simulink model "g"  (R2018b)
settings: Solver=FixedStepAuto  StartTime=0.0  StopTime=10.68  FixedStep=0.01  RelTol=1e-3
settings Model: Creator=yizha  LastModifiedBy=yizha

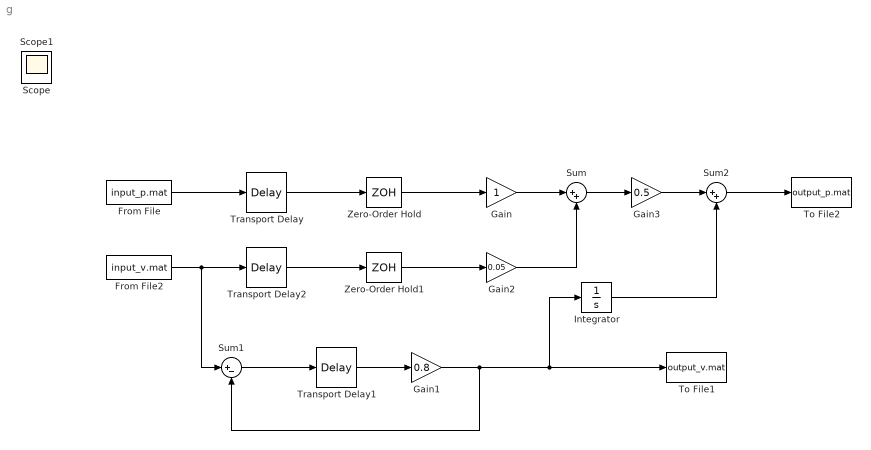
== system g ==
  From File : FromFile  FileName=input_p.mat  SampleTime=0
  From File2 : FromFile  FileName=input_v.mat  SampleTime=0
  Gain : Gain
  Gain1 : Gain  Gain=0.8
  Gain2 : Gain  Gain=0.05
  Gain3 : Gain  Gain=0.5
  Integrator : Integrator
  Sum : Sum  Inputs=|++
  Sum1 : Sum  Inputs=|+-
  Sum2 : Sum  Inputs=|++
  To File1 : ToFile  Filename=output_v.mat
  To File2 : ToFile  Filename=output_p.mat
  Transport Delay : TransportDelay  DelayTime=0.1
  Transport Delay1 : TransportDelay  DelayTime=0.1
  Transport Delay2 : TransportDelay  DelayTime=0.1
  Zero-Order Hold : ZeroOrderHold  SampleTime=0.1
  Zero-Order Hold1 : ZeroOrderHold  SampleTime=0.1
  Scope : Scope
  Scope1 : Scope
  wires:
  Sum1/1 -> Transport Delay1/1
  Transport Delay1/1 -> Gain1/1
  Gain1/1 -> Sum1/2, Integrator/1, To File1/1
  From File2/1 -> Sum1/1, Transport Delay2/1
  Transport Delay/1 -> Zero-Order Hold/1
  Gain/1 -> Sum/1
  Zero-Order Hold1/1 -> Gain2/1
  From File/1 -> Transport Delay/1
  Zero-Order Hold/1 -> Gain/1
  Transport Delay2/1 -> Zero-Order Hold1/1
  Gain2/1 -> Sum/2
  Sum2/1 -> To File2/1
  Integrator/1 -> Sum2/2
  Sum/1 -> Gain3/1
  Gain3/1 -> Sum2/1
